simulink model "powerwindow_final"  (Simulink 8.4)
settings: Solver=ode45  StartTime=0.0  StopTime=10.0  RelTol=1e-3
libraries: simulink x4
Description:
  | <HiP-HOPS_Model_Parameters><ToolVersion><Name>Matlab</Name><Number>7.14.0.739 </Number></ToolVersion><RiskTime>100000</RiskTime><OptimisationParams><MaxGenerations>100</MaxGenerations></OptimisationParams><Hazards><Hazard><Name>Unintended Move of Window</Name><Description></Description><SafetyRequirement>0</SafetyRequirement><Causes><Cause><Probability></Probability><FailureLogic>InvalidValue-power_window_control_system.control.move_up + InvalidValue-power_window_control_system.control.move_down</FailureLogic></Cause></Causes></Hazard><Hazard><Name>Pinch Detection Malfunction</Name><Description>If the system fails to detect an obstacle in the window path (i.e. a human apengage) it will can cause physical harm to the user.</Description><SafetyRequirement>0</SafetyRequirement><Causes><Cause><Probability></Probability><FailureLogic>Omission-power_window_control_system.detect_obstacle_endstop.detect_obstacle.obstacle + Comission-power_window_control_system.detect_obstacle_endstop.detect_obstacle.obstacle</FailureLogic></Cause></Causes></Hazard><Hazard><Name>Window Did Not Stop on Fully Open or Close</Name><Description>The motor should stop when the window is fully open or fully closed. This could damage the motor.</Description><SafetyRequirement>0</SafetyRequirement><Causes><Cause><Probability></Probability><FailureLogic>Comission-power_window_control_system.detect_obstacle_endstop.detect_endstop.endstop</FailureLogic></Cause></Causes></Hazard><Hazard><Name>Window Does Not Move on Request</Name><Description></Description><SafetyRequirement>0</SafetyRequirement><Causes><Cause><Probability></Probability><FailureLogic>Omission-window_system.plant.q</FailureLogic></Cause></Causes></Hazard></Hazards><AdvancedParameters></AdvancedParameters></HiP-HOPS_Model_Parameters>
settings Model: Creator=Jordan  LastModifiedBy=z2akhtar
settings DebuggingCC: FcnCallInpInsideContextMsg=EnableAllAsWarning
settings GRTTargetCC: CombineOutputUpdateFcns=on  GRTInterface=off

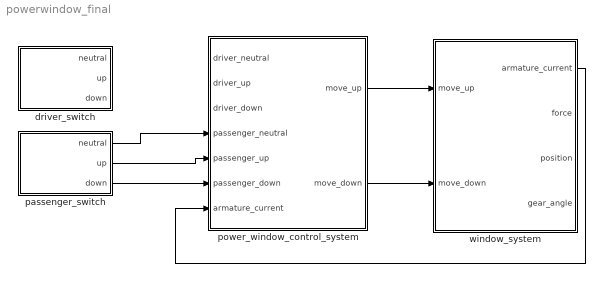
== system powerwindow_final ==
  driver_switch : Subsystem
  passenger_switch : Subsystem
  power_window_control_system : Subsystem
  window_system : Subsystem
  wires:
  passenger_switch/1(neutral) -> power_window_control_system/4(passenger_neutral)
  passenger_switch/2(up) -> power_window_control_system/5(passenger_up)
  passenger_switch/3(down) -> power_window_control_system/6(passenger_down)
  power_window_control_system/1(move_up) -> window_system/1(move_up)
  power_window_control_system/2(move_down) -> window_system/2(move_down)
  window_system/1(armature_current) -> power_window_control_system/7(armature_current)

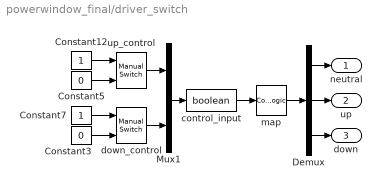
== system powerwindow_final/driver_switch ==
  Constant12 : Constant
  Constant3 : Constant  Value=0
  Constant5 : Constant  Value=0
  Constant7 : Constant
  Demux : Demux  Outputs=3
  Mux1 : Mux  Inputs=2
  control_input : DataTypeConversion  OutDataTypeStr=boolean  SaturateOnIntegerOverflow=on  RndMeth=Zero
  down_control : simulink/Signal Routing/Manual Switch  sw=0  action=0  varsize=off
  map : CombinatorialLogic  TruthTable=[1 0 0;0 0 1;0 1 0;1 0 0]
  up_control : simulink/Signal Routing/Manual Switch  sw=1  action=0  varsize=off
  neutral : Outport
  up : Outport  Port=2
  down : Outport  Port=3
  wires:
  control_input/1 -> map/1
  Constant12/1 -> up_control/1
  Constant5/1 -> up_control/2
  Constant7/1 -> down_control/1
  Constant3/1 -> down_control/2
  down_control/1 -> Mux1/2
  Mux1/1 -> control_input/1
  up_control/1 -> Mux1/1
  map/1 -> Demux/1
  Demux/1 -> neutral/1
  Demux/2 -> up/1
  Demux/3 -> down/1

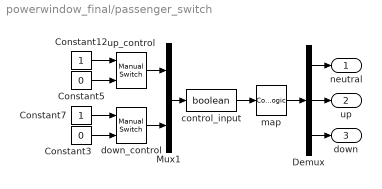
== system powerwindow_final/passenger_switch ==
  Constant12 : Constant
  Constant3 : Constant  Value=0
  Constant5 : Constant  Value=0
  Constant7 : Constant
  Demux : Demux  Outputs=3
  Mux1 : Mux  Inputs=2
  control_input : DataTypeConversion  OutDataTypeStr=boolean  SaturateOnIntegerOverflow=on  RndMeth=Zero
  down_control : simulink/Signal Routing/Manual Switch  sw=0  action=0  varsize=off
  map : CombinatorialLogic  TruthTable=[1 0 0;0 0 1;0 1 0;1 0 0]
  up_control : simulink/Signal Routing/Manual Switch  sw=0  action=0  varsize=off
  neutral : Outport
  up : Outport  Port=2
  down : Outport  Port=3
  wires:
  Demux/3 -> down/1
  Demux/2 -> up/1
  Demux/1 -> neutral/1
  map/1 -> Demux/1
  up_control/1 -> Mux1/1
  Mux1/1 -> control_input/1
  down_control/1 -> Mux1/2
  Constant3/1 -> down_control/2
  Constant7/1 -> down_control/1
  Constant5/1 -> up_control/2
  Constant12/1 -> up_control/1
  control_input/1 -> map/1

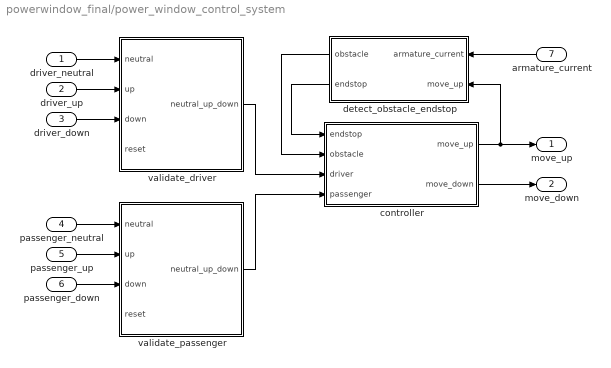
== system powerwindow_final/power_window_control_system ==
  driver_neutral : Inport
  driver_up : Inport  Port=2
  driver_down : Inport  Port=3
  passenger_neutral : Inport  Port=4
  passenger_up : Inport  Port=5
  passenger_down : Inport  Port=6
  armature_current : Inport  Port=7
  controller : Subsystem
  detect_obstacle_endstop : Subsystem
  validate_driver : Subsystem
  validate_passenger : Subsystem
  move_up : Outport
  move_down : Outport  Port=2
  wires:
  passenger_neutral/1 -> validate_passenger/1(neutral)
  passenger_up/1 -> validate_passenger/2(up)
  passenger_down/1 -> validate_passenger/3(down)
  driver_neutral/1 -> validate_driver/1(neutral)
  driver_down/1 -> validate_driver/3(down)
  armature_current/1 -> detect_obstacle_endstop/1(armature_current)
  detect_obstacle_endstop/2(endstop) -> controller/1(endstop)
  detect_obstacle_endstop/1(obstacle) -> controller/2(obstacle)
  validate_driver/1(neutral_up_down) -> controller/3(driver)
  controller/2(move_down) -> move_down/1
  controller/1(move_up) -> move_up/1, detect_obstacle_endstop/2(move_up)
  validate_passenger/1(neutral_up_down) -> controller/4(passenger)
  driver_up/1 -> validate_driver/2(up)

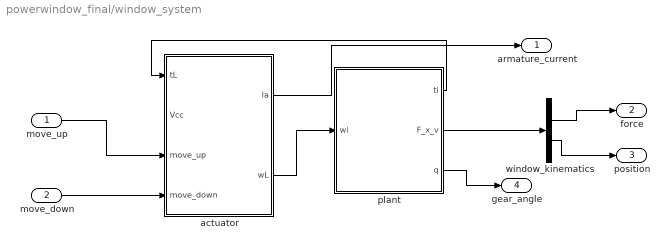
== system powerwindow_final/window_system ==
  move_up : Inport
  move_down : Inport  Port=2
  actuator : Subsystem
  plant : Subsystem
  window_kinematics : Demux  Outputs=[1,1,2,1,4]
  armature_current : Outport
  force : Outport  Port=2
  position : Outport  Port=3
  gear_angle : Outport  Port=4
  wires:
  plant/3(q) -> gear_angle/1
  plant/2(F_x_v) -> window_kinematics/1
  window_kinematics/2 -> force/1
  window_kinematics/4 -> position/1
  actuator/1(la) -> armature_current/1
  plant/1(ti) -> actuator/1(tL)
  move_up/1 -> actuator/3(move_up)
  move_down/1 -> actuator/4(move_down)
  actuator/2(wL) -> plant/1(wi)

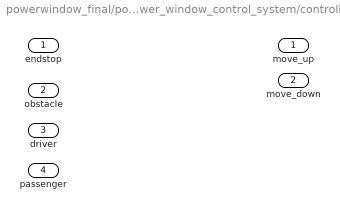
== system powerwindow_final/power_window_control_system/controller ==
  endstop : Inport
  obstacle : Inport  Port=2
  driver : Inport  Port=3
  passenger : Inport  Port=4
  move_up : Outport
  move_down : Outport  Port=2

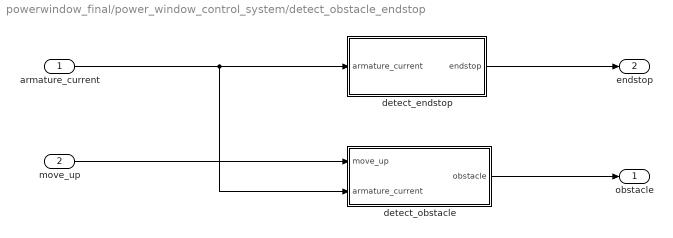
== system powerwindow_final/power_window_control_system/detect_obstacle_endstop ==
  armature_current : Inport
  move_up : Inport  Port=2
  detect_endstop : Subsystem
  detect_obstacle : Subsystem
  obstacle : Outport
  endstop : Outport  Port=2
  wires:
  detect_obstacle/1(obstacle) -> obstacle/1
  detect_endstop/1(endstop) -> endstop/1
  move_up/1 -> detect_obstacle/1(move_up)
  armature_current/1 -> detect_endstop/1(armature_current), detect_obstacle/2(armature_current)

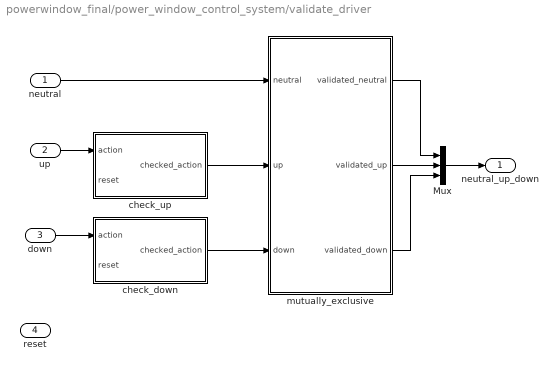
== system powerwindow_final/power_window_control_system/validate_driver ==
  neutral : Inport
  up : Inport  Port=2
  down : Inport  Port=3
  reset : Inport  Port=4
  Mux : Mux  Inputs=3
  check_down : Subsystem
  check_up : Subsystem
  mutually_exclusive : Subsystem
  neutral_up_down : Outport
  wires:
  Mux/1 -> neutral_up_down/1
  check_up/1(checked_action) -> mutually_exclusive/2(up)
  neutral/1 -> mutually_exclusive/1(neutral)
  up/1 -> check_up/1(action)
  down/1 -> check_down/1(action)
  mutually_exclusive/1(validated_neutral) -> Mux/1
  mutually_exclusive/2(validated_up) -> Mux/2
  check_down/1(checked_action) -> mutually_exclusive/3(down)
  mutually_exclusive/3(validated_down) -> Mux/3

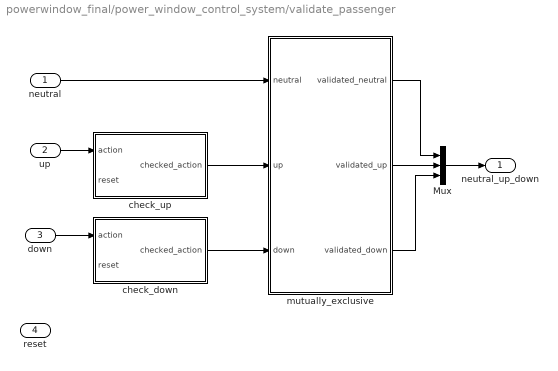
== system powerwindow_final/power_window_control_system/validate_passenger ==
  neutral : Inport
  up : Inport  Port=2
  down : Inport  Port=3
  reset : Inport  Port=4
  Mux : Mux  Inputs=3
  check_down : Subsystem
  check_up : Subsystem
  mutually_exclusive : Subsystem
  neutral_up_down : Outport
  wires:
  Mux/1 -> neutral_up_down/1
  check_up/1(checked_action) -> mutually_exclusive/2(up)
  neutral/1 -> mutually_exclusive/1(neutral)
  up/1 -> check_up/1(action)
  down/1 -> check_down/1(action)
  mutually_exclusive/1(validated_neutral) -> Mux/1
  mutually_exclusive/2(validated_up) -> Mux/2
  mutually_exclusive/3(validated_down) -> Mux/3
  check_down/1(checked_action) -> mutually_exclusive/3(down)

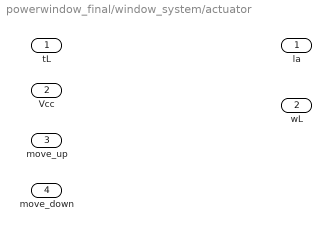
== system powerwindow_final/window_system/actuator ==
  tL : Inport
  Vcc : Inport  Port=2
  move_up : Inport  Port=3
  move_down : Inport  Port=4
  la : Outport
  wL : Outport  Port=2

== system powerwindow_final/window_system/plant ==
  wi : Inport
  ti : Outport
  F_x_v : Outport  Port=2
  q : Outport  Port=3

== system powerwindow_final/power_window_control_system/detect_obstacle_endstop/detect_endstop ==
  armature_current : Inport
  endstop : Outport

== system powerwindow_final/power_window_control_system/detect_obstacle_endstop/detect_obstacle ==
  move_up : Inport
  armature_current : Inport  Port=2
  obstacle : Outport

== system powerwindow_final/power_window_control_system/validate_driver/check_down ==
  action : Inport
  reset : Inport  Port=2
  allow_action : Logic
  overrule : Logic  Operator=NOT
  checked_action : Outport
  wires:
  reset/1 -> overrule/1
  allow_action/1 -> checked_action/1
  action/1 -> allow_action/1
  overrule/1 -> allow_action/2

== system powerwindow_final/power_window_control_system/validate_driver/check_up ==
  action : Inport
  reset : Inport  Port=2
  allow_action : Logic
  overrule : Logic  Operator=NOT
  checked_action : Outport
  wires:
  overrule/1 -> allow_action/2
  action/1 -> allow_action/1
  allow_action/1 -> checked_action/1
  reset/1 -> overrule/1

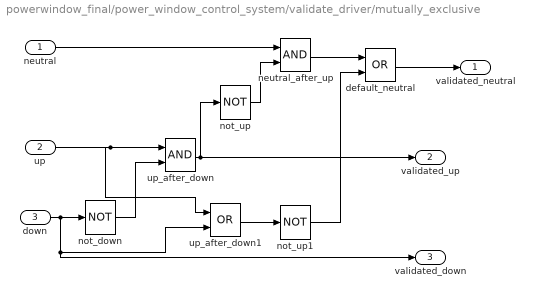
== system powerwindow_final/power_window_control_system/validate_driver/mutually_exclusive ==
  neutral : Inport
  up : Inport  Port=2
  down : Inport  Port=3
  default_neutral : Logic  Operator=OR
  neutral_after_up : Logic
  not_down : Logic  Operator=NOT
  not_up : Logic  Operator=NOT
  not_up1 : Logic  Operator=NOT
  up_after_down : Logic
  up_after_down1 : Logic  Operator=OR
  validated_neutral : Outport
  validated_up : Outport  Port=2
  validated_down : Outport  Port=3
  wires:
  not_down/1 -> up_after_down/2
  up_after_down/1 -> not_up/1, validated_up/1
  not_up/1 -> neutral_after_up/2
  down/1 -> not_down/1, up_after_down1/2, validated_down/1
  neutral/1 -> neutral_after_up/1
  up/1 -> up_after_down/1, up_after_down1/1
  up_after_down1/1 -> not_up1/1
  neutral_after_up/1 -> default_neutral/1
  default_neutral/1 -> validated_neutral/1
  not_up1/1 -> default_neutral/2

== system powerwindow_final/power_window_control_system/validate_passenger/check_down ==
  action : Inport
  reset : Inport  Port=2
  allow_action : Logic
  overrule : Logic  Operator=NOT
  checked_action : Outport
  wires:
  reset/1 -> overrule/1
  allow_action/1 -> checked_action/1
  action/1 -> allow_action/1
  overrule/1 -> allow_action/2

== system powerwindow_final/power_window_control_system/validate_passenger/check_up ==
  action : Inport
  reset : Inport  Port=2
  allow_action : Logic
  overrule : Logic  Operator=NOT
  checked_action : Outport
  wires:
  overrule/1 -> allow_action/2
  action/1 -> allow_action/1
  allow_action/1 -> checked_action/1
  reset/1 -> overrule/1

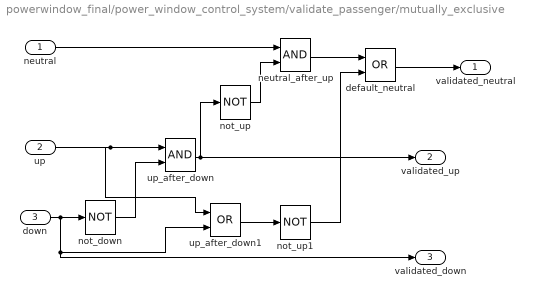
== system powerwindow_final/power_window_control_system/validate_passenger/mutually_exclusive ==
  neutral : Inport
  up : Inport  Port=2
  down : Inport  Port=3
  default_neutral : Logic  Operator=OR
  neutral_after_up : Logic
  not_down : Logic  Operator=NOT
  not_up : Logic  Operator=NOT
  not_up1 : Logic  Operator=NOT
  up_after_down : Logic
  up_after_down1 : Logic  Operator=OR
  validated_neutral : Outport
  validated_up : Outport  Port=2
  validated_down : Outport  Port=3
  wires:
  not_down/1 -> up_after_down/2
  up_after_down/1 -> not_up/1, validated_up/1
  not_up/1 -> neutral_after_up/2
  down/1 -> not_down/1, up_after_down1/2, validated_down/1
  neutral/1 -> neutral_after_up/1
  up/1 -> up_after_down/1, up_after_down1/1
  up_after_down1/1 -> not_up1/1
  neutral_after_up/1 -> default_neutral/1
  default_neutral/1 -> validated_neutral/1
  not_up1/1 -> default_neutral/2
